simulink model "Apartado_A"  (R2024b)
settings: Solver=VariableStepAuto  StartTime=0.0  StopTime=200e-3  MaxStep=1e-4  RelTol=1e-3
InitFcn:
  | clc
  | clear all
StopFcn:
  | ApartadoA
libraries: spsDiodeLib x6, spsCurrentMeasurementLib x4, spsParallelRLCBranchLib x4, spsRMSLib x2, spsThreePhaseProgrammableVoltageSourceLib x1, spsVoltageMeasurementLib x1, sps_lib x1
settings Model: Creator=javier  LastModifiedBy=javier

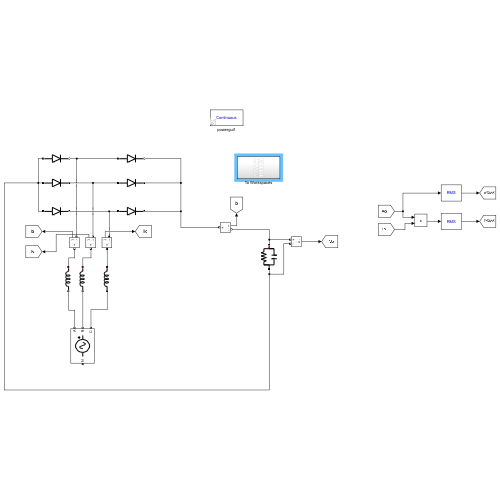
[thumbnail: Simulink's stored preview of the top-level diagram]
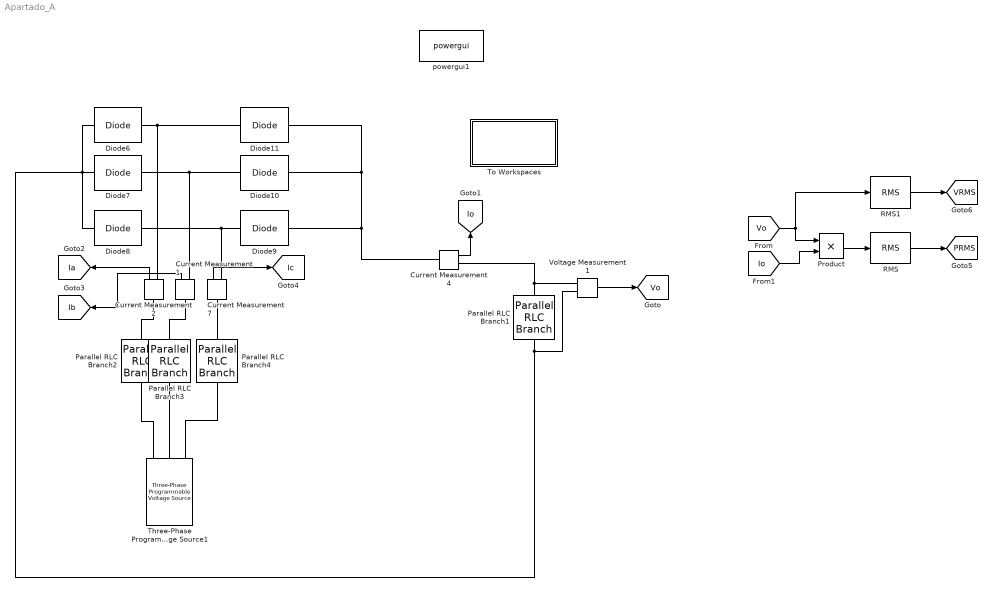
== system Apartado_A ==
  Current Measurement{1..2,4,7} (4 alike) : spsCurrentMeasurementLib/Current Measurement  PhasorSimulation=off  OutputType=Complex  PSBequivalent=0
  Diode{6..11} (6 alike) : spsDiodeLib/Diode  Ron=0.001  Lon=0  Vf=0.8  IC=0  UseSnubber=0  Rs=500  Cs=250e-9  Measurements=off
  Parallel RLC Branch1 : spsParallelRLCBranchLib/Parallel RLC Branch  LConnTagsString=a  RConnTagsString=__new0  BranchType=RC  Resistance=30  Inductance=1e-3  SetiL0=off  InitialCurrent=0  Capacitance=10e-3  Setx0=off  InitialVoltage=0  Measurements=None
  Parallel RLC Branch2 : spsParallelRLCBranchLib/Parallel RLC Branch  LConnTagsString=a  RConnTagsString=__new0  BranchType=L  Resistance=30  Inductance=5e-3  SetiL0=off  InitialCurrent=0  Capacitance=1e-6  Setx0=off  InitialVoltage=0  Measurements=None
  Parallel RLC Branch3 : spsParallelRLCBranchLib/Parallel RLC Branch  LConnTagsString=a  RConnTagsString=__new0  BranchType=L  Resistance=30  Inductance=5e-3  SetiL0=off  InitialCurrent=0  Capacitance=1e-6  Setx0=off  InitialVoltage=0  Measurements=None
  Parallel RLC Branch4 : spsParallelRLCBranchLib/Parallel RLC Branch  LConnTagsString=a  RConnTagsString=__new0  BranchType=L  Resistance=30  Inductance=5e-3  SetiL0=off  InitialCurrent=0  Capacitance=1e-6  Setx0=off  InitialVoltage=0  Measurements=None
  Product : Product
  RMS : spsRMSLib/RMS  TrueRMS=on  Freq=60  RMSInit=120  Ts=0
  RMS1 : spsRMSLib/RMS  TrueRMS=on  Freq=60  RMSInit=120  Ts=0
  Three-Phase Programmable Voltage Source1 : spsThreePhaseProgrammableVoltageSourceLib/Three-Phase Programmable Voltage Source  PositiveSequence="[400  0 50]"  VariationEntity=None  VariationType=Table of time-amplitude pairs  VariationTypeAlt=Step  VariationStep=0.5  VariationRate=10  VariationMagnitude=0.3  VariationFrequency=2  VariationTiming=[1 2]  VariationPhaseA=off  Amplitudes=[1 0.8 1.2 1.0]  TimeValues=[0 0.1 0.15 0.2]  HarmonicGeneration=off  HarmonicA=[3 0.2 -25 0]  HarmonicB=[2 0.15 35 2]  Timing="[0.05  3]"  BusType=swing  Pref=0  Qref=0  Qmin=-inf  Qmax=inf
  To Workspaces : Subsystem
  Voltage Measurement1 : spsVoltageMeasurementLib/Voltage Measurement  PhasorSimulation=off  OutputType=Complex  PSBequivalent=0
  powergui1 : sps_lib/powergui  Priority=1  SimulationMode=Continuous  SampleTime=50e-6  frequency=60  Iterations=50  frequencyindice=50  Pbase=100e6  ErrMax=1e-4  UnitsV=kV  UnitsW=MW  buscounter=0  FunctionMessages=off  echomessages=off  EnableUseOfTLC=off  CurrentSourceSwitches=off  DisableSnubberDevices=on  DisableRonSwitches=off  DisableVfSwitches=off  DisplayEquations=off  AutomaticDiscreteSolvers=off  SolverType=Tustin/Backward Euler (TBE)  Interpol=off  ExternalGateDelay=off  methode=off  Ts=100  x0status=blocks  SPID=on  SwTol=0  HookPort=off  NonlinearTolerance=1e-4  nMaxIteration=100  ContinueOnMaxIteration=off  RestoreLinks=warning  ResistiveCurrentMeasurement=off  Frange=[0:2:500]  Ylog=off  Xlog=on  ShowGrid=off  save=off  variable=ZData  structure=0  ZoomFFT=off  StartTime=0.0  cycles=1  DisplayStyle=1  fundamental=60  FreqAxis=off  MaxFrequency=1000  frequencyindicesteady=1  RmsSteady=1  display=off
  tag scope: Ia=global, Ib=global, Ic=global, Io=global, PRMS=global, VRMS=global, Vo=global
  wires:
  Voltage Measurement1/1 -> [Vo]
  Current Measurement4/1 -> [Io]
  Current Measurement7/1 -> [Ic]
  [Vo] -> RMS1/1, Product/1
  [Io] -> Product/2
  Product/1 -> RMS/1
  RMS/1 -> [PRMS]
  RMS1/1 -> [VRMS]
  Current Measurement2/1 -> [Ia]
  Current Measurement1/1 -> [Ib]
  connections:
  Diode6/LConn1 -- Voltage Measurement1/LConn2 -- Parallel RLC Branch1/RConn1 -- Diode8/LConn1 -- Diode7/LConn1
  Diode10/RConn1 -- Diode11/RConn1 -- Current Measurement4/LConn1 -- Diode9/RConn1
  Parallel RLC Branch1/LConn1 -- Current Measurement4/RConn1 -- Voltage Measurement1/LConn1
  Diode7/RConn1 -- Diode10/LConn1 -- Current Measurement1/RConn1
  Current Measurement7/RConn1 -- Diode8/RConn1 -- Diode9/LConn1
  Diode6/RConn1 -- Current Measurement2/RConn1 -- Diode11/LConn1
  Parallel RLC Branch2/RConn1 -- Three-Phase Programmable Voltage Source1/RConn1
  Three-Phase Programmable Voltage Source1/RConn2 -- Parallel RLC Branch3/RConn1
  Three-Phase Programmable Voltage Source1/RConn3 -- Parallel RLC Branch4/RConn1
  Current Measurement7/LConn1 -- Parallel RLC Branch4/LConn1
  Current Measurement1/LConn1 -- Parallel RLC Branch3/LConn1
  Current Measurement2/LConn1 -- Parallel RLC Branch2/LConn1

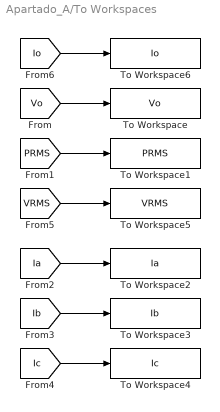
== system Apartado_A/To Workspaces ==
  To Workspace : ToWorkspace  VariableName=Vo  SaveFormat=Timeseries  SampleTime=-1
  To Workspace1 : ToWorkspace  VariableName=PRMS  SaveFormat=Timeseries  SampleTime=-1
  To Workspace2 : ToWorkspace  VariableName=Ia  SaveFormat=Timeseries  SampleTime=-1
  To Workspace3 : ToWorkspace  VariableName=Ib  SaveFormat=Timeseries  SampleTime=-1
  To Workspace4 : ToWorkspace  VariableName=Ic  SaveFormat=Timeseries  SampleTime=-1
  To Workspace5 : ToWorkspace  VariableName=VRMS  SaveFormat=Timeseries  SampleTime=-1
  To Workspace6 : ToWorkspace  VariableName=Io  SaveFormat=Timeseries  SampleTime=-1
  wires:
  [Ic] -> To Workspace4/1
  [Vo] -> To Workspace/1
  [Ia] -> To Workspace2/1
  [Ib] -> To Workspace3/1
  [PRMS] -> To Workspace1/1
  [VRMS] -> To Workspace5/1
  [Io] -> To Workspace6/1
